simulink subsystem "PLL"  (R2022b)
settings: Solver=VariableStepAuto  StartTime=0.0  StopTime=10.0  RelTol=1e-3
settings Model: Creator=Ali-Laptop  LastModifiedBy=Ali-Laptop

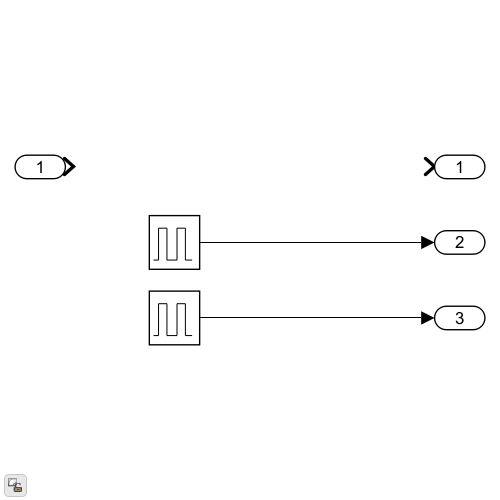
[thumbnail: Simulink's stored preview of the top-level diagram]
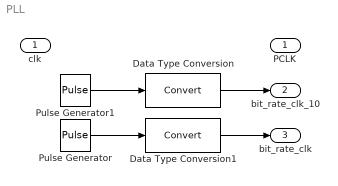
== system PLL ==
  clk : Inport
  Data Type Conversion : DataTypeConversion  SaturateOnIntegerOverflow=off  RndMeth=Floor
  Data Type Conversion1 : DataTypeConversion  SaturateOnIntegerOverflow=off  RndMeth=Floor
  Pulse Generator : DiscretePulseGenerator  PulseType=Time based  Period=1/5e9  PulseWidth=50
  Pulse Generator1 : DiscretePulseGenerator  PulseType=Time based  Period=1/500e6  PulseWidth=50
  PCLK : Outport
  bit_rate_clk_10 : Outport  Port=2
  bit_rate_clk : Outport  Port=3
  wires:
  Pulse Generator/1 -> Data Type Conversion1/1
  Pulse Generator1/1 -> Data Type Conversion/1
  Data Type Conversion/1 -> bit_rate_clk_10/1
  Data Type Conversion1/1 -> bit_rate_clk/1
